simulink model "Linux_test_create_AM_data"  (R2021b)
settings: Solver=VariableStepAuto  StartTime=0.0  StopTime=20  FixedStep=5e-07  RelTol=1e-3
libraries: commanapbnd3 x1, commchan3 x1, dspvision x1
settings Model: Creator=caccolillo  LastModifiedBy=caccolillo

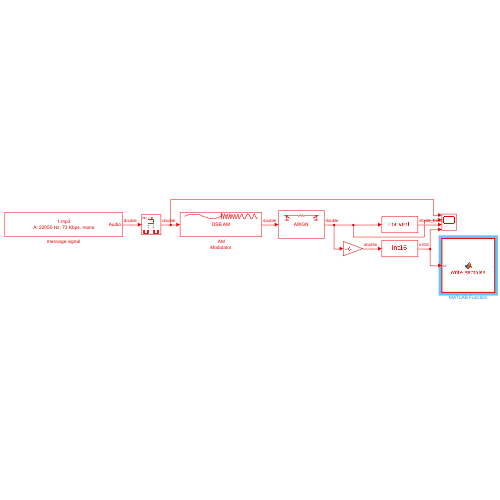
[thumbnail: Simulink's stored preview of the top-level diagram]
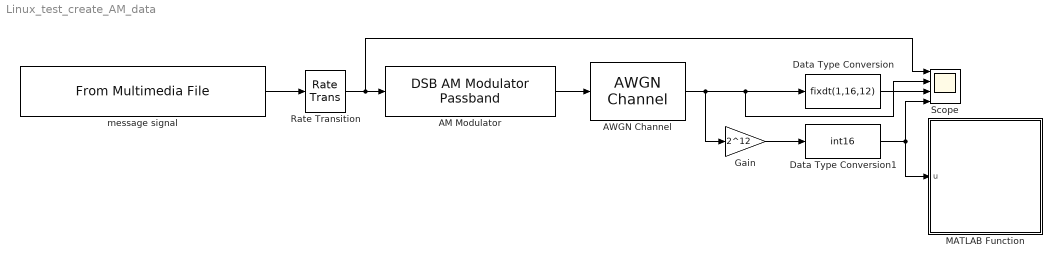
== system Linux_test_create_AM_data ==
  " AM Modulator " : commanapbnd3/DSB AM Modulator Passband  Fc=500000  Ph=0  Offset=1
      settings: SourceProductBaseCode=CM
  AWGN Channel : commchan3/AWGN Channel  InputProcessing=Columns as channels (frame based)  seed=67  noiseMode="Signal to noise ratio  (Eb/No)"  EbNodB=75  EsNodB=10  SNRdB=10  bitsPerSym=1  Ps=1  Tsym=1  variance=1
  Data Type Conversion : DataTypeConversion  OutDataTypeStr=fixdt(1,16,12)
  Data Type Conversion1 : DataTypeConversion  OutDataTypeStr=int16
  Gain : Gain  Gain=2^12
  MATLAB Function : MATLAB Function  TreatAsAtomicUnit=on
  Rate Transition : RateTransition  Deterministic=off
  Scope : Scope  NumInputPorts=4
  message signal : dspvision/From Multimedia File  inputFilename=/home/caccolillo/hilbert_transform_am/audio/1.mp3  readRange=[1 Inf]  loop=on  numPlays=inf  outputStreams=Audio only  videoDataType=single  audioDataType=double  inheritSampleTime=on  userDefinedSampleTime=5.0E-7  noAudioOutput=off  isIntensityVideo=off  fourcc=RGB  colorVideoFormat=Separate color signals  outputEOF=off  dataOrg=Column-major  audioFrameSize=1  computeAudioFrameSize=off  outSamplingMode=Frame based
  wires:
  Rate Transition/1 -> " AM Modulator "/1, Scope/1
  Gain/1 -> Data Type Conversion1/1
  " AM Modulator "/1 -> AWGN Channel/1
  Data Type Conversion/1 -> Scope/3
  message signal/1 -> Rate Transition/1
  Data Type Conversion1/1 -> MATLAB Function/1(u), Scope/4
  AWGN Channel/1 -> Data Type Conversion/1, Scope/2, Gain/1

== matlab function Linux_test_create_AM_data/MATLAB Function ==
  data: u input
function write_samples(u)
%#codegen
persistent fid
if isempty(fid)
    fid = fopen('samples.txt','w');
end
fprintf(fid, '%d\n', int16(u));
